simulink model "controlador_predictivo_neural_network"  (R2019a)
settings: Solver=VariableStepAuto  StartTime=0.0  StopTime=120  RelTol=1e-3
undefined symbols (not defined in the file or in its folder): now
libraries: neural x1
settings Model: Creator=cmparedes  LastModifiedBy=cmparedes

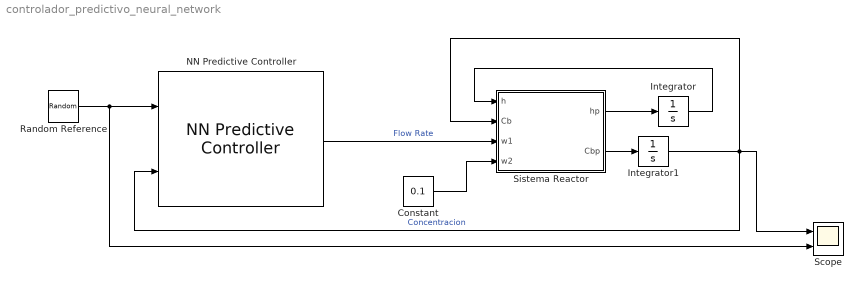
== system controlador_predictivo_neural_network ==
  Constant : Constant  Value=0.1
  Integrator : Integrator  InitialCondition=30
  Integrator1 : Integrator  InitialCondition=22
  NN Predictive Controller : neural/Control Systems/NN Predictive Controller  epochs=200  minp=0.10091272597214517859  maxp=3.9815589106203668202  mint=20.055666720010147941  maxt=3.9815589106203668202  Normalize=0  IW=[-0.049811616913444628496 0.22894308605421676006;0.61789986002975205714 0.83485382000229990673;0.10225225127105846967 -0.081165021289146557781;0.0014641228140105015752 -0.0014831306633601426797;-0.0038752965948436286434 0.0086322063017781891503;-0.62935718104396254358 -1.9286438739971323297;-5.1564235113029015523 -3.8232485136062579478]  LW1_2=[-0.18858273569261996272 0.25141020686163273457;2.1169897643992312553 0.95970732754464438408;0.37174091633579064986 0.87238838052312295268;0.4497338298899676845 -0.22700989114173469874;1.5791081754188662778 -0.33528511323257975674;0.95662522610183187144 0.34516370051425132592;1.3347111869917103188 0.39044087056713727701]  LW2_1=[7.6584520045275032984 -0.49842634204520619434 0.086682461993220896734 4.4331319751378179816 0.088298751818836451744 0.094930613029329813379 0.0001401453577100638477]  B1=[33.637911929897214236;-28.291037867366629399;-24.608677038731560316;-4.7687773345256871949;-28.703573754912198979;-14.078096280391681816;-17.51623613398087187]  B2=14.157812346537713921  max_i_int=20  min_i_int=5  limit_output=1  max_output=23  min_output=20  Use_Previous_Weights=1  N2=7  Nu=2  Ts=0.2  rho=0.05  alpha=0.001  csrchfun=csrchbac  maxiter=2  S1=7  Ni=2  Nj=2  sim_file=cstr  trainfun=trainlm  Use_validation=1  Use_Testing=1  max_i=4  min_i=0  sam_training=8000
      settings: SourceProductName=MATLAB Runtime - Deep Learning Toolbox  SourceProductBaseCode=Missing
  Random Reference : UniformRandomNumber  Minimum=20  Maximum=23  Seed=round(now)  SampleTime=20
  Scope : Scope  NumInputPorts=2
  Sistema Reactor : MATLAB Function  TreatAsAtomicUnit=on
  wires:
  Sistema Reactor/1(hp) -> Integrator/1
  Integrator/1 -> Sistema Reactor/1(h)
  Sistema Reactor/2(Cbp) -> Integrator1/1
  Integrator1/1 -> Scope/1, Sistema Reactor/2(Cb), NN Predictive Controller/2  "Concentracion"
  NN Predictive Controller/1 -> Sistema Reactor/3(w1)  "Flow Rate"
  Constant/1 -> Sistema Reactor/4(w2)
  Random Reference/1 -> Scope/2, NN Predictive Controller/1

== matlab function controlador_predictivo_neural_network/Sistema Reactor ==
  data: h input; hp output; Cb input; w1 input; w2 input; Cbp output
function [hp,Cbp] = fcn(h,Cb,w1,w2)

Cb1=24.9;
Cb2=0.1;
k1=1;
k2=1;

hp = w1+w2-0.2*sqrt(h);
Cbp=(Cb1-Cb)*w1/h+(Cb2-Cb)*w2/h-k1*Cb/((1+k2*Cb)^2);
